simulink model "ProgramandoEmBlocos"  (R2021b)
settings: Solver=VariableStepAuto  StartTime=0.0  StopTime=10.0  RelTol=1e-3
settings Model: Creator=20.00387-0  LastModifiedBy=20.00387-0

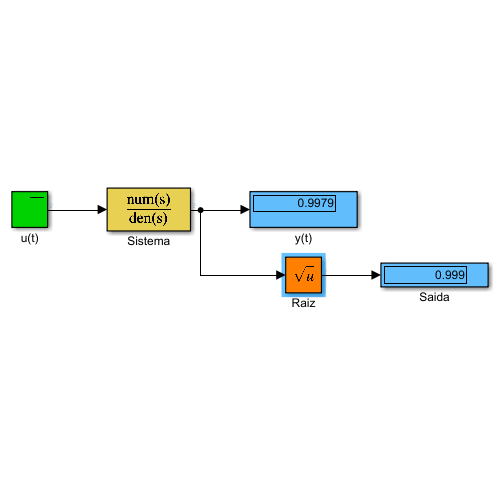
[thumbnail: Simulink's stored preview of the top-level diagram]
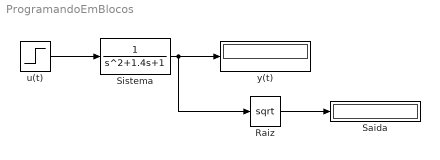
== system ProgramandoEmBlocos ==
  Raiz : Sqrt  SaturateOnIntegerOverflow=on
  Saida : Display
  Sistema : TransferFcn  Denominator=[1 1.4 1]
  u(t) : Step  SampleTime=0
  y(t) : Display
  wires:
  u(t)/1 -> Sistema/1
  Sistema/1 -> y(t)/1, Raiz/1
  Raiz/1 -> Saida/1
